simulink model "SystemARMAX"  (Simulink 6.3)
settings: Solver=FixedStepDiscrete  StartTime=0.0  StopTime=tend  RelTol=1e-3
values from neighbouring files (symbols this model uses):
  c1o = 0.99    [ZADANIE_1_2.m]    (also in ZADANIE_2_1.m = 0; Zad_1_1.m = 0; Zad_1_1_8_kolorowe.m; Zad_2_1_zapominanie.m = 0)
  Td = 1500    [ZADANIE_1_2.m]    (also in ZADANIE_2_1.m = 500; Zad_1_1.m; Zad_1_1_8_kolorowe.m; Zad_2_1_zapominanie.m = 500)
  Tp = 0.1    [ZADANIE_1_2.m]    (also in ZADANIE_2_1.m; Zad_1_1.m; Zad_1_1_8_kolorowe.m; Zad_2_1_zapominanie.m)
libraries: simulink x4
settings Model: LastModifiedBy=Maciej

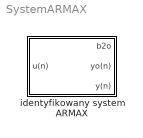
== system SystemARMAX ==
  identyfikowany system ARMAX : Subsystem

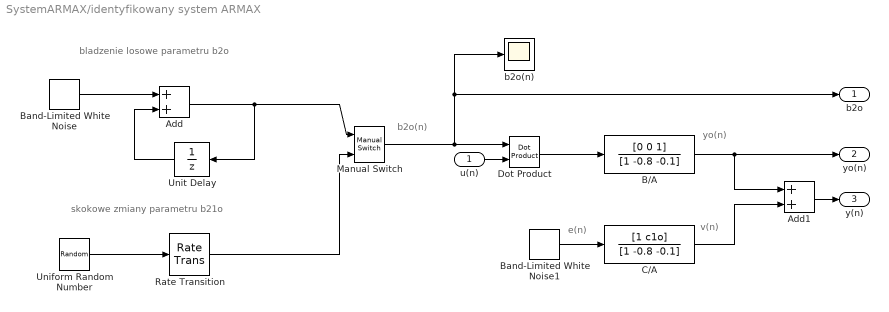
== system SystemARMAX/identyfikowany system ARMAX ==
  note: e(n)
  note: v(n)
  note: yo(n)
  note: b2o(n)
  note: skokowe zmiany parametru b21o
  note: bladzenie losowe parametru b2o
  u(n) : Inport
  Add : Sum  OutScaling=2^-10
  Add1 : Sum  OutScaling=2^-10
  B/A : DiscreteFilter  Numerator=[0 0 1]  Denominator=[1 -0.8 -0.1]  SampleTime=Tp
  Band-Limited White Noise : simulink/Sources/Band-Limited White Noise  Cov=[0.00001*Tp]  Ts=Tp  seed=[23341]
  Band-Limited White Noise1 : simulink/Sources/Band-Limited White Noise  Cov=[0.001*Tp]  Ts=Tp  seed=[23341]
  C/A : DiscreteFilter  Numerator=[1 c1o]  Denominator=[1 -0.8 -0.1]  SampleTime=Tp
  Dot Product : simulink/Math Operations/Dot Product  InputSameDT=on  OutDataType=sfix(16)  OutScaling=2^-10  DoSatur=off
  Manual Switch : simulink/Signal Routing/Manual Switch  sw=1  action=0
  Rate Transition : RateTransition  X0=0.5  OutPortSampleTime=Tp
  Uniform Random Number : UniformRandomNumber  Minimum=0.1  Maximum=0.8  Seed=2  SampleTime=Td
  Unit Delay : UnitDelay  Orientation=left  SampleTime=Tp
  b2o(n) : Scope
  b2o : Outport
  yo(n) : Outport  Port=2
  y(n) : Outport  Port=3
  wires:
  Band-Limited White Noise/1 -> Add/1
  Add/1 -> Unit Delay/1, Manual Switch/1
  Unit Delay/1 -> Add/2
  Uniform Random Number/1 -> Rate Transition/1
  Rate Transition/1 -> Manual Switch/2
  Manual Switch/1 -> Dot Product/1, b2o/1, b2o(n)/1
  Dot Product/1 -> B/A/1
  C/A/1 -> Add1/2
  B/A/1 -> Add1/1, yo(n)/1
  Band-Limited White Noise1/1 -> C/A/1
  u(n)/1 -> Dot Product/2
  Add1/1 -> y(n)/1
